simulink model "mdaqdemo_pil"  (R2013a)
settings: Solver=FixedStepDiscrete  StartTime=0.0  StopTime=inf  FixedStep=0.1  RelTol=1e-3
settings Model: Creator=peselnikmg  LastModifiedBy=skibool
settings DataIOCC: SignalLoggingSaveFormat=ModelDataLogs
settings OptimizationCC: OptimizeModelRefInitCode=on  LifeSpan=1
settings HardwareCC: ProdBitPerLong=40  ProdLargestAtomicInteger=Integer  ProdIntDivRoundTo=Zero  ProdEndianess=LittleEndian  ProdHWDeviceType=Texas Instruments->C6000
settings RTWCC: SystemTargetFile=microdaq.tlc  TemplateMakefile=microdaq.tmf  PostCodeGenCommand=microdaq_postcodegen(buildInfo)  Description=MicroDAQ Real-Time Measurement System  GenerateReport=on  ProcessScript=microdaq_make_rtw_hook  IncludeHyperlinkInReport=on  LaunchReport=on
settings CodeAppCC: IgnoreCustomStorageClasses=off
settings STFCustomTargetCC: CodeReplacementLibrary=TI C674x  CombineOutputUpdateFcns=on  ERTCustomFileBanners=on  SupportContinuousTime=off  SupportNonInlinedSFcns=off  MATLABClassNameForMDSCustomization=Simulink.SoftwareTarget.ERTCustomization  SystemTargetFile=microdaq.tlc
settings ERTTargetCC: CodeReplacementLibrary=TI C674x  GenerateSampleERTMain=off  ParMdlRefBuildCompliant=off  CompOptLevelCompliant=off  ConcurrentExecutionCompliant=off  ERTFirstTimeCompliant=off  ModelStepFunctionPrototypeControlCompliant=off  CPPClassGenCompliant=off  ERTCustomFileTemplate=microdaq_main.tlc

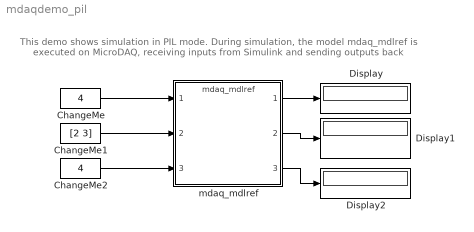
== system mdaqdemo_pil ==
  note: This demo shows simulation in PIL mode.
      | During simulation, the model mdaq_mdlref is executed on MicroDAQ,
      | receiving inputs from Simulink and sending outputs back
  ChangeMe : Constant  Value=4  OutDataTypeStr=Inherit: Inherit via back propagation
  ChangeMe1 : Constant  Value=[2 3]  OutDataTypeStr=Inherit: Inherit via back propagation
  ChangeMe2 : Constant  Value=4  OutDataTypeStr=Inherit: Inherit via back propagation
  Display : Display
  Display1 : Display
  Display2 : Display
  mdaq_mdlref : ModelReference  ModelNameDialog=mdaq_mdlref  SimulationMode=Processor-in-the-loop (PIL)  ModelReferenceVersion=1.21  CopyOfModelName=mdaq_mdlref  DefaultDataLogging=on
  wires:
  ChangeMe/1 -> mdaq_mdlref/1
  mdaq_mdlref/1 -> Display/1
  mdaq_mdlref/2 -> Display1/1
  mdaq_mdlref/3 -> Display2/1
  ChangeMe1/1 -> mdaq_mdlref/2
  ChangeMe2/1 -> mdaq_mdlref/3
